simulink model "gm_sampleModel1911_4_sub"  (R2023a)
settings: Solver=VariableStepAuto  StartTime=0.0  StopTime=10.0  RelTol=1e-3
libraries: simulink x3
settings Model: Creator=user1  LastModifiedBy=user1
settings OptimizationCC: BlockReduction=off  ConditionallyExecuteInputs=off
settings DebuggingCC: InheritedTsInSrcMsg=none

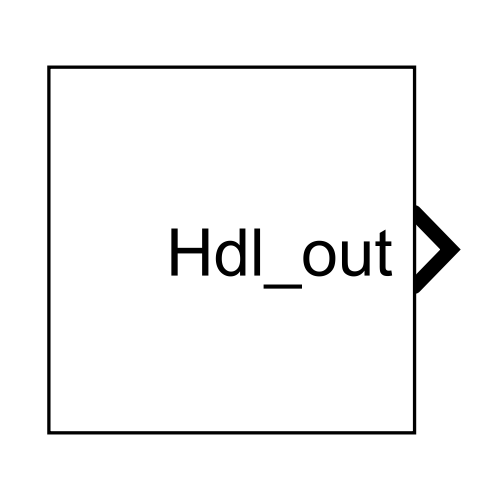
[thumbnail: Simulink's stored preview of the top-level diagram]
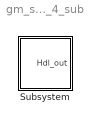
== system gm_sampleModel1911_4_sub ==
  Subsystem : Subsystem

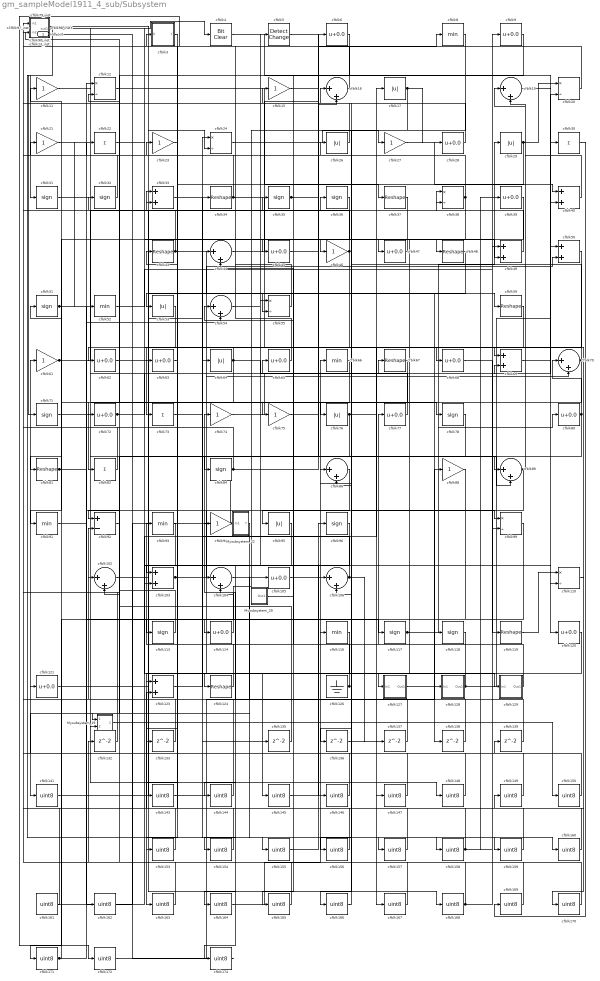
== system gm_sampleModel1911_4_sub/Subsystem ==
  Mysubsystem_19 : Subsystem
  Mysubsystem_22 : Subsystem
  Mysubsystem_29 : Subsystem
  cfblk101_inst : Subsystem
  cfblk{16,19,44,54,70,86,89,102,104,106} (10 alike) : Sum  Inputs=|++  OutDataTypeStr=uint8
  cfblk{33,40,49..50,69,103,123} (7 alike) : Sum  OutDataTypeStr=uint8
  cfblk{6,9,28,39,45,47,62..63,65,68,72,77,80,105,114,120..121} (17 alike) : Bias  Bias=0.0  SaturateOnIntegerOverflow=off
  cfblk108_inst : Subsystem
  cfblk10_inst : Subsystem
  cfblk{11,15,21,23,27,46,61,74..75,88,94} (11 alike) : Gain  OutDataTypeStr=uint8
  cfblk{12,20,24,38,55,99,110} (7 alike) : Product  Inputs=*/  OutDataTypeStr=uint8  RndMeth=Zero  SaturateOnIntegerOverflow=on
  cfblk111_inst : Subsystem
  cfblk{31..32,35..36,51,71,78,84,96,113,117..118} (12 alike) : Signum
  cfblk115_inst : Subsystem
  cfblk{8,52,66,91,93,116} (6 alike) : MinMax  OutDataTypeStr=uint8
  cfblk{34,37,43,48,59,67,81,119,124} (9 alike) : Reshape
  cfblk126 : Ground
  cfblk127 : Subsystem
  cfblk128 : Subsystem
  cfblk129 : Subsystem
  cfblk{132..133,135..139} (7 alike) : Delay  SampleTime=1
  cfblk13_inst : Subsystem
  cfblk{141,143..150,153..172,174} (30 alike) : DataTypeConversion  OutDataTypeStr=uint8  SaturateOnIntegerOverflow=off  RndMeth=Floor
  cfblk{17,26,29,53,64,76,95} (7 alike) : Abs  OutDataTypeStr=uint8  SaturateOnIntegerOverflow=off
  cfblk{22,30,73,82} (4 alike) : Sum  Inputs=+  OutDataTypeStr=uint8
  cfblk3 : Subsystem  mask(Detect Fall Nonpositive){vinit=double(0), InputProcessing=Elements as channels (sample based), OutDataTypeStr=uint8}
      mask prompts: vinit "Simulink:masks:InitialCondition_MP"; InputProcessing "Simulink:masks:InputProcessing_MP"; OutDataTypeStr "Simulink:masks:OutputDataType_MP"
      mask help: Simulink:masks:DetectFallNonpositive_MD
      mask init:
      | InputProcessing = 'Elements as channels (sample based)';
      | OutDataTypeStr = 'uint8';
      | vinit = double(0);
      mask TypeOptions InputProcessing: Simulink:masks:ColumnsAsChannelsFrameBased | Simulink:masks:ElementsAsChannelsSampleBased
      mask TypeOptions OutDataTypeStr: Simulink:masks:uint8 | Simulink:masks:boolean
      mask Display: fprintf('U <= 0\n&  NOT\nU/z <= 0')
  cfblk4 : simulink/Logic and Bit Operations/Bit Clear  iBit=0
      settings: LibrarySourceBlock=|
      | hdlsllib/Logic and Bit
      | Operations/Bit Clear
  cfblk5 : simulink/Logic and Bit Operations/Detect Change  vinit=0  OutDataTypeStr=uint8
      settings: LibrarySourceBlock=|
      | hdlsllib/Logic and Bit
      | Operations/Detect
      | Change
  cfblk79_inst : Subsystem
  cfblk90_inst : Subsystem
  cfblk92 : Sum  Inputs=+-  OutDataTypeStr=uint8
  cfblk97_inst : Subsystem
  cfblk98_inst : Subsystem
  Hdl_out : Outport  OutDataTypeStr=uint8  SampleTime=1
  wires:
  Mysubsystem_19/1(Out1) -> cfblk150/1
  Mysubsystem_22/1(Y) -> cfblk141/1
  Mysubsystem_29/1(Out1) -> cfblk65/1
  cfblk10_inst/1(out1) -> cfblk155/1
  cfblk101_inst/1(out1) -> cfblk149/1, cfblk24/2, Mysubsystem_19/2(In2)
  cfblk102/1 -> cfblk168/1
  cfblk103/1 -> cfblk70/2, cfblk50/2
  cfblk104/1 -> cfblk160/1
  cfblk105/1 -> cfblk66/1
  cfblk106/1 -> cfblk24/1, cfblk137/1
  cfblk108_inst/1(out1) -> cfblk48/1
  cfblk11/1 -> cfblk148/1
  cfblk110/1 -> cfblk170/1
  cfblk111_inst/1(out1) -> cfblk59/1, cfblk157/1
  cfblk113/1 -> cfblk115_inst/2(in2)
  cfblk114/1 -> cfblk74/1
  cfblk115_inst/1(out1) -> cfblk31/1
  cfblk116/1 -> cfblk163/1
  cfblk117/1 -> cfblk80/1, cfblk29/1
  cfblk118/1 -> cfblk77/1
  cfblk119/1 -> cfblk110/1
  cfblk12/1 -> cfblk37/1
  cfblk120/1 -> cfblk124/1
  cfblk121/1 -> cfblk36/1
  cfblk123/1 -> cfblk34/1
  cfblk124/1 -> cfblk64/1
  cfblk126/1 -> cfblk54/1, cfblk44/2
  cfblk127/1(Out1) -> cfblk128/1(In1)
  cfblk128/1(Out1) -> cfblk16/1, cfblk20/2
  cfblk129/1(Out1) -> cfblk93/1
  cfblk13_inst/1(out1) -> cfblk145/1
  cfblk132/1 -> cfblk90_inst/2(in2)
  cfblk133/1 -> cfblk92/2
  cfblk135/1 -> cfblk12/2
  cfblk136/1 -> cfblk159/1
  cfblk137/1 -> cfblk98_inst/1(in1)
  cfblk138/1 -> cfblk104/1
  cfblk139/1 -> cfblk101_inst/1(in1)
  cfblk141/1 -> cfblk17/1
  cfblk143/1 -> cfblk105/1
  cfblk144/1 -> cfblk3/1(U)
  cfblk145/1 -> cfblk106/1
  cfblk146/1 -> cfblk13_inst/1(in1)
  cfblk147/1 -> cfblk13_inst/2(in2)
  cfblk148/1 -> cfblk61/1
  cfblk149/1 -> cfblk11/1
  cfblk15/1 -> cfblk78/1
  cfblk150/1 -> cfblk139/1
  cfblk153/1 -> cfblk101_inst/2(in2)
  cfblk154/1 -> cfblk23/1
  cfblk155/1 -> cfblk96/1
  cfblk156/1 -> cfblk10_inst/1(in1)
  cfblk157/1 -> cfblk10_inst/2(in2)
  cfblk158/1 -> cfblk9/1, cfblk39/1, cfblk123/2
  cfblk159/1 -> cfblk33/1
  cfblk16/1 -> cfblk172/1
  cfblk160/1 -> cfblk33/2
  cfblk161/1 -> cfblk108_inst/2(in2)
  cfblk162/1 -> cfblk94/1
  cfblk163/1 -> cfblk79_inst/1(in1)
  cfblk164/1 -> cfblk116/1
  cfblk165/1 -> cfblk79_inst/2(in2)
  cfblk166/1 -> cfblk86/1
  cfblk167/1 -> cfblk86/2
  cfblk168/1 -> cfblk99/2, cfblk132/1
  cfblk169/1 -> cfblk102/1
  cfblk17/1 -> cfblk28/1, cfblk106/2, cfblk104/2
  cfblk170/1 -> cfblk102/2
  cfblk171/1 -> cfblk54/2, cfblk121/1
  cfblk172/1 -> cfblk88/1
  cfblk174/1 -> Hdl_out/1
  cfblk19/1 -> cfblk30/1
  cfblk20/1 -> cfblk115_inst/1(in1)
  cfblk21/1 -> cfblk162/1
  cfblk22/1 -> cfblk46/1
  cfblk23/1 -> cfblk153/1
  cfblk24/1 -> cfblk27/1
  cfblk26/1 -> cfblk108_inst/1(in1)
  cfblk27/1 -> cfblk40/1
  cfblk28/1 -> cfblk15/1
  cfblk29/1 -> cfblk154/1, cfblk103/1, cfblk20/1
  cfblk3/1(Y) -> cfblk143/1
  cfblk30/1 -> cfblk169/1
  cfblk31/1 -> cfblk135/1
  cfblk32/1 -> cfblk12/1
  cfblk33/1 -> cfblk158/1
  cfblk34/1 -> cfblk98_inst/2(in2), cfblk147/1
  cfblk35/1 -> cfblk6/1, cfblk49/2, cfblk47/1
  cfblk36/1 -> cfblk113/1
  cfblk37/1 -> cfblk95/1
  cfblk38/1 -> cfblk90_inst/1(in1), cfblk127/1(In1)
  cfblk39/1 -> cfblk81/1
  cfblk4/1 -> cfblk120/1
  cfblk40/1 -> cfblk19/2
  cfblk43/1 -> cfblk97_inst/2(in2), cfblk138/1
  cfblk44/1 -> cfblk8/1
  cfblk45/1 -> cfblk68/1
  cfblk46/1 -> cfblk114/1, cfblk111_inst/1(in1)
  cfblk47/1 -> cfblk45/1
  cfblk48/1 -> cfblk53/1
  cfblk49/1 -> cfblk38/1
  cfblk5/1 -> cfblk89/2
  cfblk50/1 -> cfblk133/1
  cfblk51/1 -> cfblk76/1, cfblk22/1
  cfblk52/1 -> cfblk49/1
  cfblk53/1 -> cfblk73/1
  cfblk54/1 -> cfblk5/1
  cfblk55/1 -> cfblk21/1
  cfblk59/1 -> cfblk164/1
  cfblk6/1 -> cfblk55/2
  cfblk61/1 -> cfblk69/2, cfblk35/1
  cfblk62/1 -> cfblk44/1
  cfblk63/1 -> cfblk43/1
  cfblk64/1 -> cfblk63/1, cfblk146/1, cfblk82/1
  cfblk65/1 -> cfblk111_inst/2(in2)
  cfblk66/1 -> cfblk91/1
  cfblk67/1 -> cfblk136/1
  cfblk68/1 -> cfblk119/1
  cfblk69/1 -> cfblk50/1
  cfblk70/1 -> cfblk62/1, cfblk26/1, cfblk156/1
  cfblk71/1 -> cfblk118/1
  cfblk72/1 -> cfblk67/1, cfblk129/1(In1)
  cfblk73/1 -> cfblk89/1
  cfblk74/1 -> cfblk40/2
  cfblk75/1 -> cfblk16/2
  cfblk76/1 -> cfblk167/1, Mysubsystem_19/1(In1)
  cfblk77/1 -> cfblk55/1
  cfblk78/1 -> cfblk92/1
  cfblk79_inst/1(out1) -> cfblk69/1
  cfblk8/1 -> cfblk75/1
  cfblk80/1 -> cfblk84/1, cfblk70/1
  cfblk81/1 -> cfblk117/1, cfblk99/1
  cfblk82/1 -> cfblk97_inst/1(in1)
  cfblk84/1 -> cfblk51/1, cfblk38/2, Mysubsystem_22/1(In1)
  cfblk86/1 -> cfblk165/1
  cfblk88/1 -> cfblk171/1
  cfblk89/1 -> cfblk19/1, cfblk166/1
  cfblk9/1 -> cfblk72/1
  cfblk90_inst/1(out1) -> cfblk71/1
  cfblk91/1 -> cfblk52/1
  cfblk92/1 -> cfblk32/1
  cfblk93/1 -> cfblk103/2
  cfblk94/1 -> cfblk161/1
  cfblk95/1 -> cfblk144/1
  cfblk96/1 -> cfblk123/1
  cfblk97_inst/1(out1) -> cfblk110/2
  cfblk98_inst/1(out1) -> cfblk4/1
  cfblk99/1 -> cfblk174/1

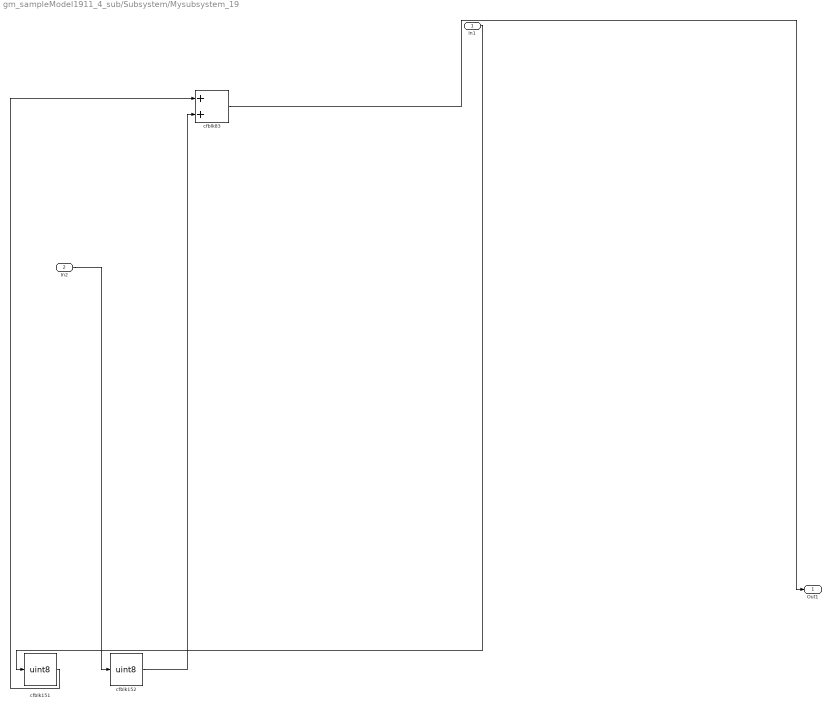
== system gm_sampleModel1911_4_sub/Subsystem/Mysubsystem_19 ==
  In1 : Inport  OutDataTypeStr=uint8  PortDimensions=1  SampleTime=1
  In2 : Inport  Port=2  OutDataTypeStr=uint8  PortDimensions=1  SampleTime=1
  cfblk151 : DataTypeConversion  OutDataTypeStr=uint8  SaturateOnIntegerOverflow=off  RndMeth=Floor
  cfblk152 : DataTypeConversion  OutDataTypeStr=uint8  SaturateOnIntegerOverflow=off  RndMeth=Floor
  cfblk83 : Sum
  Out1 : Outport  SampleTime=1
  wires:
  In1/1 -> cfblk151/1
  In2/1 -> cfblk152/1
  cfblk151/1 -> cfblk83/1
  cfblk152/1 -> cfblk83/2
  cfblk83/1 -> Out1/1

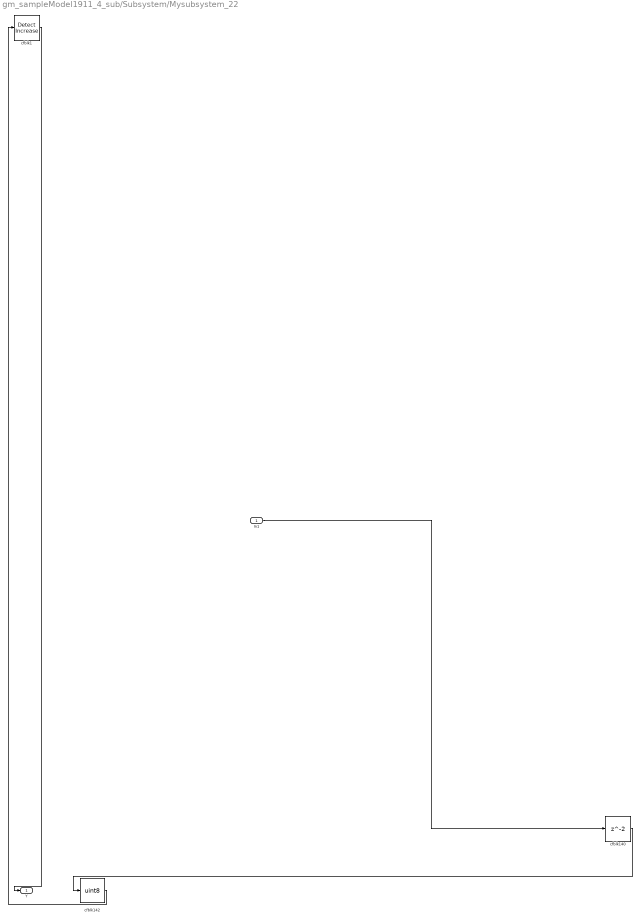
== system gm_sampleModel1911_4_sub/Subsystem/Mysubsystem_22 ==
  In1 : Inport  OutDataTypeStr=uint8  PortDimensions=1  SampleTime=1
  cfblk1 : simulink/Logic and Bit Operations/Detect Increase  vinit=0.0  OutDataTypeStr=boolean
      settings: LibrarySourceBlock=|
      | hdlsllib/Logic and Bit
      | Operations/Detect
      | Increase
  cfblk140 : Delay  SampleTime=1
  cfblk142 : DataTypeConversion  OutDataTypeStr=uint8  SaturateOnIntegerOverflow=off  RndMeth=Floor
  Y : Outport  SampleTime=1
  wires:
  In1/1 -> cfblk140/1
  cfblk1/1 -> Y/1
  cfblk140/1 -> cfblk142/1
  cfblk142/1 -> cfblk1/1

== system gm_sampleModel1911_4_sub/Subsystem/Mysubsystem_29 ==
  cfblk125 : Ground
  Out1 : Outport  SampleTime=1
  wires:
  cfblk125/1 -> Out1/1

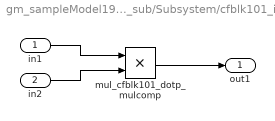
== system gm_sampleModel1911_4_sub/Subsystem/cfblk101_inst ==
  in1 : Inport  OutDataTypeStr=uint8  SampleTime=1
  in2 : Inport  Port=2  OutDataTypeStr=uint8  SampleTime=1
  mul_cfblk101_dotp_mulcomp : Product  Inputs=**  OutDataTypeStr=uint8  SampleTime=1
  out1 : Outport  OutDataTypeStr=uint8  SampleTime=1
  wires:
  in1/1 -> mul_cfblk101_dotp_mulcomp/1
  in2/1 -> mul_cfblk101_dotp_mulcomp/2
  mul_cfblk101_dotp_mulcomp/1 -> out1/1

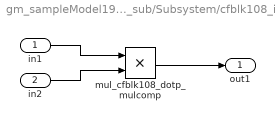
== system gm_sampleModel1911_4_sub/Subsystem/cfblk108_inst ==
  in1 : Inport  OutDataTypeStr=uint8  SampleTime=1
  in2 : Inport  Port=2  OutDataTypeStr=uint8  SampleTime=1
  mul_cfblk108_dotp_mulcomp : Product  Inputs=**  OutDataTypeStr=uint8  SampleTime=1
  out1 : Outport  OutDataTypeStr=uint8  SampleTime=1
  wires:
  in1/1 -> mul_cfblk108_dotp_mulcomp/1
  in2/1 -> mul_cfblk108_dotp_mulcomp/2
  mul_cfblk108_dotp_mulcomp/1 -> out1/1

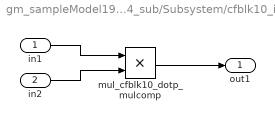
== system gm_sampleModel1911_4_sub/Subsystem/cfblk10_inst ==
  in1 : Inport  OutDataTypeStr=uint8  SampleTime=1
  in2 : Inport  Port=2  OutDataTypeStr=uint8  SampleTime=1
  mul_cfblk10_dotp_mulcomp : Product  Inputs=**  OutDataTypeStr=uint8  SampleTime=1
  out1 : Outport  OutDataTypeStr=uint8  SampleTime=1
  wires:
  in1/1 -> mul_cfblk10_dotp_mulcomp/1
  in2/1 -> mul_cfblk10_dotp_mulcomp/2
  mul_cfblk10_dotp_mulcomp/1 -> out1/1

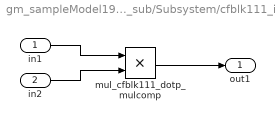
== system gm_sampleModel1911_4_sub/Subsystem/cfblk111_inst ==
  in1 : Inport  OutDataTypeStr=uint8  SampleTime=1
  in2 : Inport  Port=2  OutDataTypeStr=uint8  SampleTime=1
  mul_cfblk111_dotp_mulcomp : Product  Inputs=**  OutDataTypeStr=uint8  SampleTime=1
  out1 : Outport  OutDataTypeStr=uint8  SampleTime=1
  wires:
  in1/1 -> mul_cfblk111_dotp_mulcomp/1
  in2/1 -> mul_cfblk111_dotp_mulcomp/2
  mul_cfblk111_dotp_mulcomp/1 -> out1/1

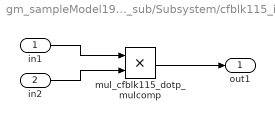
== system gm_sampleModel1911_4_sub/Subsystem/cfblk115_inst ==
  in1 : Inport  OutDataTypeStr=uint8  SampleTime=1
  in2 : Inport  Port=2  OutDataTypeStr=uint8  SampleTime=1
  mul_cfblk115_dotp_mulcomp : Product  Inputs=**  OutDataTypeStr=uint8  SampleTime=1
  out1 : Outport  OutDataTypeStr=uint8  SampleTime=1
  wires:
  in1/1 -> mul_cfblk115_dotp_mulcomp/1
  in2/1 -> mul_cfblk115_dotp_mulcomp/2
  mul_cfblk115_dotp_mulcomp/1 -> out1/1

== system gm_sampleModel1911_4_sub/Subsystem/cfblk127 ==
  In1 : Inport  OutDataTypeStr=uint8  PortDimensions=1  SampleTime=1
  Out1 : Outport  SampleTime=1
  wires:
  In1/1 -> Out1/1

== system gm_sampleModel1911_4_sub/Subsystem/cfblk128 ==
  In1 : Inport  OutDataTypeStr=uint8  PortDimensions=1  SampleTime=1
  Out1 : Outport  SampleTime=1
  wires:
  In1/1 -> Out1/1

== system gm_sampleModel1911_4_sub/Subsystem/cfblk129 ==
  In1 : Inport  OutDataTypeStr=uint8  PortDimensions=1  SampleTime=1
  Out1 : Outport  SampleTime=1
  wires:
  In1/1 -> Out1/1

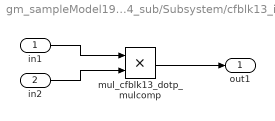
== system gm_sampleModel1911_4_sub/Subsystem/cfblk13_inst ==
  in1 : Inport  OutDataTypeStr=uint8  SampleTime=1
  in2 : Inport  Port=2  OutDataTypeStr=uint8  SampleTime=1
  mul_cfblk13_dotp_mulcomp : Product  Inputs=**  OutDataTypeStr=uint8  SampleTime=1
  out1 : Outport  OutDataTypeStr=uint8  SampleTime=1
  wires:
  in1/1 -> mul_cfblk13_dotp_mulcomp/1
  in2/1 -> mul_cfblk13_dotp_mulcomp/2
  mul_cfblk13_dotp_mulcomp/1 -> out1/1

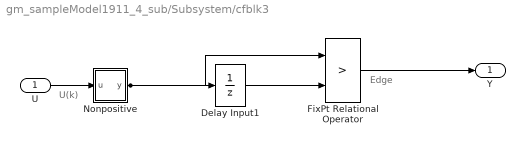
== system gm_sampleModel1911_4_sub/Subsystem/cfblk3 ==
  note: U(k)
  note: Edge
  U : Inport  OutDataTypeStr=uint8  SampleTime=1
  Delay Input1 : UnitDelay  Description=Store in Global RAM  DisableCoverage=on  InitialCondition=vinit  SampleTime=-1  HasFrameUpgradeWarning=on
  FixPt Relational Operator : RelationalOperator  Operator=>  OutDataTypeStr=fixdt(0, 8)  ZeroCross=off  InputSameDT=off
  Nonpositive : Subsystem  mask(Compare To Zero){relop=<=, OutDataTypeStr=boolean, ZeroCross=off}
      mask prompts: relop "Simulink:masks:Operator_MP"; OutDataTypeStr "Simulink:masks:OutputDataType_MP"; ZeroCross "Simulink:masks:EnableZerocrossingDetection_MP"
      mask help: Simulink:masks:CompareToZero_MD
      mask init:
      | OutDataTypeStr = 'boolean';
      | ZeroCross = 'off';
      | blkName = 'sampleModel1911_4_sub/Subsystem/cfblk3/Nonpositive';
      | relop = '<=';
      | setValue = 'boolean';
      mask TypeOptions relop: == | ~= | < | <= | >= | >
      mask TypeOptions OutDataTypeStr: Simulink:masks:uint8 | Simulink:masks:boolean
      mask Callback ZeroCross: sl('zeroCrossEnable', gcbh);
      mask Display: disp([relop,' 0'])
  Y : Outport  SampleTime=1
  wires:
  U/1 -> Nonpositive/1(u)
  Delay Input1/1 -> FixPt Relational Operator/2
  FixPt Relational Operator/1 -> Y/1
  Nonpositive/1(y) -> FixPt Relational Operator/1, Delay Input1/1

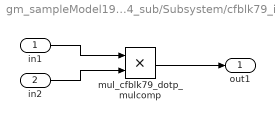
== system gm_sampleModel1911_4_sub/Subsystem/cfblk79_inst ==
  in1 : Inport  OutDataTypeStr=uint8  SampleTime=1
  in2 : Inport  Port=2  OutDataTypeStr=uint8  SampleTime=1
  mul_cfblk79_dotp_mulcomp : Product  Inputs=**  OutDataTypeStr=uint8  SampleTime=1
  out1 : Outport  OutDataTypeStr=uint8  SampleTime=1
  wires:
  in1/1 -> mul_cfblk79_dotp_mulcomp/1
  in2/1 -> mul_cfblk79_dotp_mulcomp/2
  mul_cfblk79_dotp_mulcomp/1 -> out1/1

== system gm_sampleModel1911_4_sub/Subsystem/cfblk90_inst ==
  in1 : Inport  OutDataTypeStr=uint8  SampleTime=1
  in2 : Inport  Port=2  OutDataTypeStr=uint8  SampleTime=1
  mul_cfblk90_dotp_mulcomp : Product  Inputs=**  OutDataTypeStr=uint8  SampleTime=1
  out1 : Outport  OutDataTypeStr=uint8  SampleTime=1
  wires:
  in1/1 -> mul_cfblk90_dotp_mulcomp/1
  in2/1 -> mul_cfblk90_dotp_mulcomp/2
  mul_cfblk90_dotp_mulcomp/1 -> out1/1

== system gm_sampleModel1911_4_sub/Subsystem/cfblk97_inst ==
  in1 : Inport  OutDataTypeStr=uint8  SampleTime=1
  in2 : Inport  Port=2  OutDataTypeStr=uint8  SampleTime=1
  mul_cfblk97_dotp_mulcomp : Product  Inputs=**  OutDataTypeStr=uint8  SampleTime=1
  out1 : Outport  OutDataTypeStr=uint8  SampleTime=1
  wires:
  in1/1 -> mul_cfblk97_dotp_mulcomp/1
  in2/1 -> mul_cfblk97_dotp_mulcomp/2
  mul_cfblk97_dotp_mulcomp/1 -> out1/1

== system gm_sampleModel1911_4_sub/Subsystem/cfblk98_inst ==
  in1 : Inport  OutDataTypeStr=uint8  SampleTime=1
  in2 : Inport  Port=2  OutDataTypeStr=uint8  SampleTime=1
  mul_cfblk98_dotp_mulcomp : Product  Inputs=**  OutDataTypeStr=uint8  SampleTime=1
  out1 : Outport  OutDataTypeStr=uint8  SampleTime=1
  wires:
  in1/1 -> mul_cfblk98_dotp_mulcomp/1
  in2/1 -> mul_cfblk98_dotp_mulcomp/2
  mul_cfblk98_dotp_mulcomp/1 -> out1/1

== system gm_sampleModel1911_4_sub/Subsystem/cfblk3/Nonpositive ==
  u : Inport  OutDataTypeStr=uint8  SampleTime=1
  Compare : RelationalOperator  Operator=<=  OutDataTypeStr=boolean  ZeroCross=off
  Constant : Constant  DisableCoverage=on  Value=0  OutDataTypeStr=Inherit: Inherit via back propagation  SampleTime=-1  PreserveConstantTs=on
  y : Outport  SampleTime=1
  wires:
  u/1 -> Compare/1
  Compare/1 -> y/1
  Constant/1 -> Compare/2
